simulink model "schema_sistema"  (Simulink 7.6)
settings: Solver=ode45  StartTime=0.0  StopTime=10.0  RelTol=1e-3
values from neighbouring files (symbols this model uses):
  A = [2 3;4 1]    [controllo1_BUONO.m]    (also in controllo2.m = [0 1;-k/m -h/m])
  B = [1;0]    [controllo1_BUONO.m]    (also in controllo2.m = [0;1/m])
  C = [1 0]    [controllo1_BUONO.m]    (also in controllo2.m)
  D = 0    [controllo1_BUONO.m]    (also in controllo2.m)
  ueq = 1    [controllo1_BUONO.m]    (also in controllo2.m = 3)
  x0 = [1;1]    [controllo1_BUONO.m]    (also in controllo2.m = [1;0])
libraries: simulink x1
settings Model: Creator=professore  LastModifiedBy=patrizio

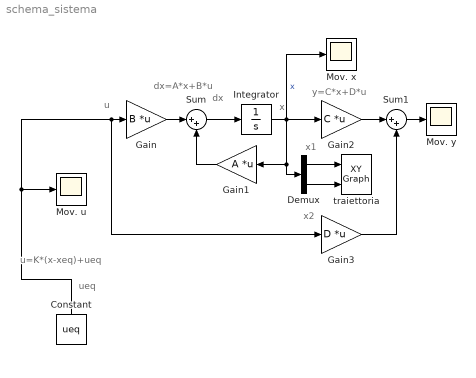
== system schema_sistema ==
  note: dx=A*x+B*u
  note: y=C*x+D*u
  note: u=K*(x-xeq)+ueq
  note: dx
  note: x
  note: u
  note: ueq
  note: x1
  note: x2
  Constant : Constant  Value=ueq
  Demux : Demux  Outputs=2
  Gain : Gain  Gain=B  Multiplication=Matrix(K*u)
  Gain1 : Gain  Gain=A  Multiplication=Matrix(K*u)
  Gain2 : Gain  Gain=C  Multiplication=Matrix(K*u)
  Gain3 : Gain  Gain=D  Multiplication=Matrix(K*u)
  Integrator : Integrator  InitialCondition=x0
  Mov. u : Scope
      settings: SaveName=ScopeData2
  Mov. x : Scope
  Mov. y : Scope
  Sum : Sum  Inputs=|++
  Sum1 : Sum  Inputs=|++
  traiettoria : simulink/Sinks/XY Graph  SystemSampleTime=-1  xmin=-10  xmax=10  ymin=-10  ymax=10  st=-1
  wires:
  Gain/1 -> Sum/1
  Gain1/1 -> Sum/2
  Sum/1 -> Integrator/1
  Integrator/1 -> Gain2/1, Gain1/1, Demux/1, Mov. x/1  "x"
  Gain2/1 -> Sum1/1
  Gain3/1 -> Sum1/2
  Constant/1 -> Gain/1, Gain3/1, Mov. u/1
  Sum1/1 -> Mov. y/1
  Demux/1 -> traiettoria/1
  Demux/2 -> traiettoria/2
